simulink model "simulink_demo_diagr"  (Simulink 7.5)
settings: Solver=ode45  StartTime=0.0  StopTime=10.0  RelTol=1e-3
values from neighbouring files (symbols this model uses):
  den = [1 2*csi*wn wn^2]    [simulink_demo.m]
  num = wn^2    [simulink_demo.m]
settings Model: Creator=jag  LastModifiedBy=jag
settings DebuggingCC: SolverPrmCheckMsg=none

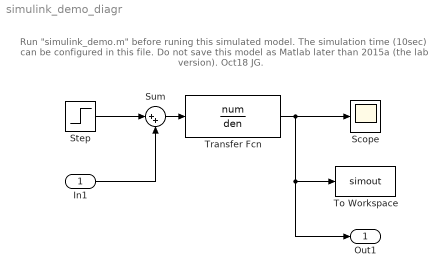
== system simulink_demo_diagr ==
  note: Run "simulink_demo.m" before runing this simulated model.
      | The simulation time (10sec) can be configured in this file.
      | Do not save this model as Matlab later than 2015a (the lab version). Oct18 JG.
  In1 : Inport  OutDataType=fixdt(1, 16)  OutScaling=2^0
  Scope : Scope
  Step : Step  SampleTime=0
  Sum : Sum  Inputs=|++  OutDataType=fixdt(1, 16)  OutScaling=2^0
  To Workspace : ToWorkspace  VariableName=simout  SampleTime=-1  SaveFormat=Structure
  Transfer Fcn : TransferFcn  Numerator=num  Denominator=den
  Out1 : Outport  OutDataType=fixdt(1, 16)  OutScaling=2^0
  wires:
  Sum/1 -> Transfer Fcn/1
  Step/1 -> Sum/1
  In1/1 -> Sum/2
  Transfer Fcn/1 -> Scope/1, Out1/1, To Workspace/1
